simulink library "crm_grc"  (R2024a)
settings: Solver=VariableStepAuto  StartTime=0.0  StopTime=10.0  RelTol=1e-3
undefined symbols (not defined in the file or in its folder): ACRM_Eta_X_rpm, ACRM_MTPAIdGen_X_rpm, ACRM_MTPAIdGen_Y_Nm, ACRM_MTPAIdGenMin_X_rpm, ACRM_MTPAIdGenMin_Y_Nm, ACRM_MTPAIdMot_X_rpm, ACRM_MTPAIdMot_Y_Nm, ACRM_MTPAIdMotMin_X_rpm, ACRM_MTPAIdMotMin_Y_Nm, ACRM_MTPAIqGen_X_rpm, ACRM_MTPAIqGen_Y_Nm, ACRM_MTPAIqGenMin_X_rpm, ACRM_MTPAIqGenMin_Y_Nm, ACRM_MTPAIqMot_X_rpm, ACRM_MTPAIqMot_Y_Nm, ACRM_MTPAIqMotMin_X_rpm, ACRM_MTPAIqMotMin_Y_Nm, ACRM_MTPVIdLimt_X_rpm, DiscIntNeverNeededParam, ENUM_MOTMOD_DISCHARGE, GRC_FAKE_SAMPLE_TIME, KCRM_AtSweep_deg_ovrdflg, KCRM_AtSweep_deg_ovrdval, KCRM_AtSwFWThd_V, KCRM_AtSwStep_ms, KCRM_AtSwThetaStep_deg, KCRM_bRstDebugOverSpd_null, KCRM_BusCurFil_null, KCRM_CurDebugSwt_null, KCRM_CurTqCmdHi_Nm, KCRM_CurTqCmdLo_Nm, KCRM_DcHiBatLDerat_V, KCRM_DcHiBatLLim_V, KCRM_DynoDeratingFiltFac_null, KCRM_FWCEnable_null, KCRM_FWCKi_null, KCRM_FWCKp_null, KCRM_grdIsThetaRampDown_C, KCRM_grdIsThetaRampUp_C, KCRM_IdCmdFilCoeff_null, KCRM_IdCmdMaxLimt_A, KCRM_IdqMapVolHi_V, KCRM_IdqMapVolLo_V, KCRM_IdSp_A_ovrdval, KCRM_IdSpForActvDisc_null, KCRM_IqCmdFilCoeff_null, KCRM_IqDeratingFac_null, KCRM_IqDeratingRecoverTi_ms, KCRM_IqDeratingTi_ms, KCRM_IqDerForFluxWeaken_fac, KCRM_IqSp_A_ovrdval, KCRM_IsSp_A, KCRM_MinVolOfst4FW_V, KCRM_MTPAGenSwitch_flg, KCRM_MTPAMotSwitch_flg, KCRM_MTPVSpdThd_rpm, KCRM_nDebugOverSpd_rpm, KCRM_OCSwFltNormThd_A, KCRM_PILowerLimit_null, KCRM_SpdCtlPrd_s ... (+24)
libraries: GRC_Lib x5, simulink x4
(part 1 of 2)
settings Model: Creator=FVT24180  LastModifiedBy=FVT22063

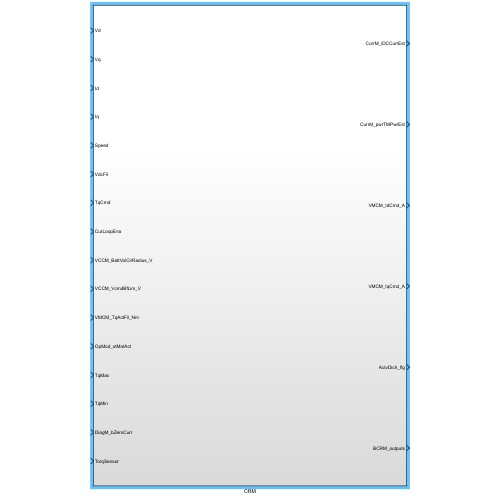
[thumbnail: Simulink's stored preview of the top-level diagram]
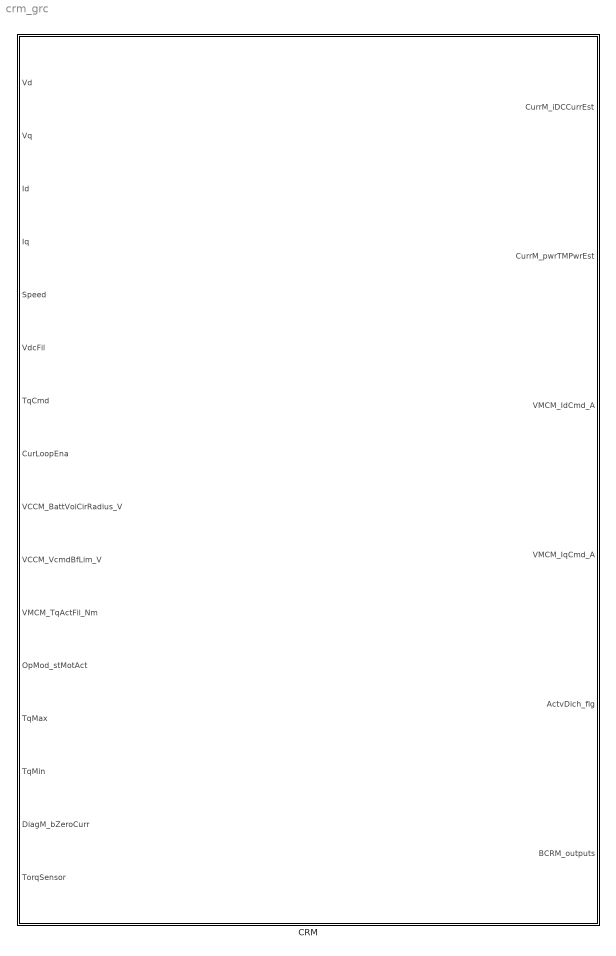
== system crm_grc ==
  CRM : Subsystem

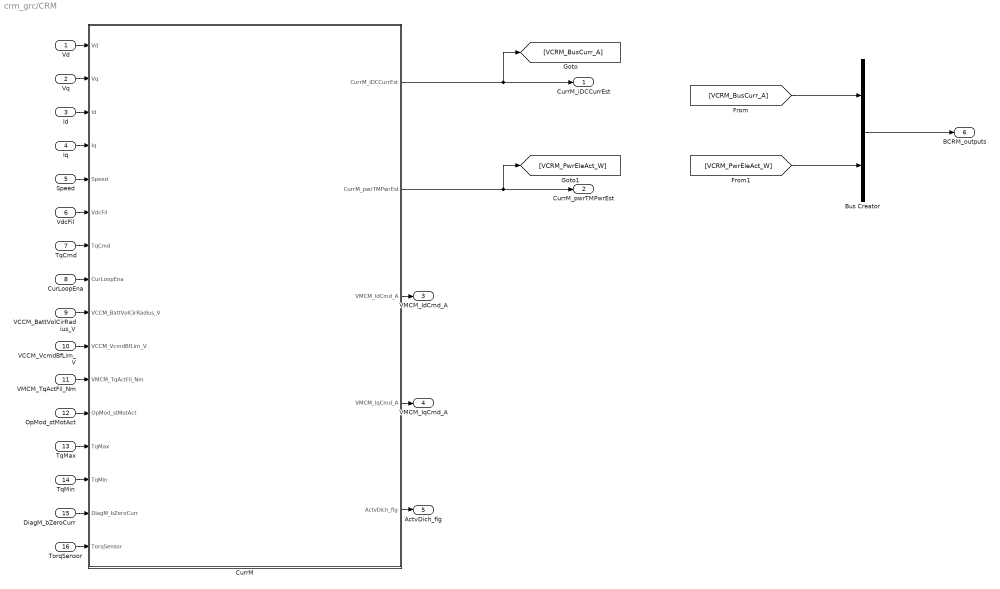
== system crm_grc/CRM ==
  "Vd " : Inport
  "Vq " : Inport  Port=2
  "Id " : Inport  Port=3
  Iq : Inport  Port=4
  "Speed " : Inport  Port=5
  "VdcFil " : Inport  Port=6
  TqCmd : Inport  Port=7
  CurLoopEna : Inport  Port=8
  VCCM_BattVolCirRadius_V : Inport  Port=9
  VCCM_VcmdBfLim_V : Inport  Port=10
  VMCM_TqActFil_Nm : Inport  Port=11
  OpMod_stMotAct : Inport  Port=12
  TqMax : Inport  Port=13
  TqMin : Inport  Port=14
  DiagM_bZeroCurr : Inport  Port=15
  "TorqSensor " : Inport  Port=16
  Bus Creator : BusCreator  Inputs=2  OutDataTypeStr=Bus: BCRM_outputs  NonVirtualBus=on
  CurrM : Subsystem
  CurrM_iDCCurrEst : Outport
  CurrM_pwrTMPwrEst : Outport  Port=2
  VMCM_IdCmd_A : Outport  Port=3
  VMCM_IqCmd_A : Outport  Port=4
  ActvDich_flg : Outport  Port=5
  BCRM_outputs : Outport  Port=6  OutDataTypeStr=Bus: BCRM_outputs
  wires:
  "Vd "/1 -> CurrM/1("Vd ")
  "Speed "/1 -> CurrM/5("Speed ")
  "Vq "/1 -> CurrM/2("Vq ")
  VCCM_VcmdBfLim_V/1 -> CurrM/10(VCCM_VcmdBfLim_V)
  CurLoopEna/1 -> CurrM/8(CurLoopEna)
  Iq/1 -> CurrM/4(Iq)
  TqMin/1 -> CurrM/14(TqMin)
  "VdcFil "/1 -> CurrM/6("VdcFil ")
  "Id "/1 -> CurrM/3("Id ")
  VMCM_TqActFil_Nm/1 -> CurrM/11(VMCM_TqActFil_Nm)
  OpMod_stMotAct/1 -> CurrM/12(OpMod_stMotAct)
  TqCmd/1 -> CurrM/7(TqCmd)
  VCCM_BattVolCirRadius_V/1 -> CurrM/9(VCCM_BattVolCirRadius_V)
  TqMax/1 -> CurrM/13(TqMax)
  CurrM/5(ActvDich_flg) -> ActvDich_flg/1
  "TorqSensor "/1 -> CurrM/16("TorqSensor ")
  DiagM_bZeroCurr/1 -> CurrM/15(DiagM_bZeroCurr)
  CurrM/4(VMCM_IqCmd_A) -> VMCM_IqCmd_A/1
  CurrM/3(VMCM_IdCmd_A) -> VMCM_IdCmd_A/1
  CurrM/1(CurrM_iDCCurrEst) -> [VCRM_BusCurr_A], CurrM_iDCCurrEst/1
  CurrM/2(CurrM_pwrTMPwrEst) -> [VCRM_PwrEleAct_W], CurrM_pwrTMPwrEst/1
  [VCRM_PwrEleAct_W] -> Bus Creator/2
  [VCRM_BusCurr_A] -> Bus Creator/1
  Bus Creator/1 -> BCRM_outputs/1

== system crm_grc/CRM/CurrM ==
  "Vd " : Inport
  "Vq " : Inport  Port=2
  "Id " : Inport  Port=3
  Iq : Inport  Port=4
  "Speed " : Inport  Port=5
  "VdcFil " : Inport  Port=6
  TqCmd : Inport  Port=7
  CurLoopEna : Inport  Port=8
  VCCM_BattVolCirRadius_V : Inport  Port=9
  VCCM_VcmdBfLim_V : Inport  Port=10
  VMCM_TqActFil_Nm : Inport  Port=11
  OpMod_stMotAct : Inport  Port=12
  TqMax : Inport  Port=13
  TqMin : Inport  Port=14
  DiagM_bZeroCurr : Inport  Port=15
  "TorqSensor " : Inport  Port=16
  EstiFun : Subsystem
  MCM : Subsystem
  CurrM_iDCCurrEst : Outport
  CurrM_pwrTMPwrEst : Outport  Port=2
  VMCM_IdCmd_A : Outport  Port=3
  VMCM_IqCmd_A : Outport  Port=4
  ActvDich_flg : Outport  Port=5
  wires:
  Iq/1 -> EstiFun/4(Iq)
  EstiFun/2(VCRM_PwrEleAct_W) -> CurrM_pwrTMPwrEst/1
  VMCM_TqActFil_Nm/1 -> MCM/6(VMCM_TqActFil_Nm)
  VCCM_BattVolCirRadius_V/1 -> MCM/4(VCCM_BattVolCirRadius_V)
  OpMod_stMotAct/1 -> MCM/7(OpMod_stMotAct)
  "Vd "/1 -> EstiFun/1("Vd ")
  CurLoopEna/1 -> MCM/3(CurLoopEna)
  "VdcFil "/1 -> EstiFun/6("VdcFil ")
  VCCM_VcmdBfLim_V/1 -> MCM/5(VCCM_VcmdBfLim_V)
  DiagM_bZeroCurr/1 -> MCM/10(DiagM_bZeroCurr)
  TqMin/1 -> MCM/9(TqMin)
  "TorqSensor "/1 -> MCM/11("TorqSensor ")
  TqMax/1 -> MCM/8(TqMax)
  TqCmd/1 -> MCM/1(TqCmd)
  MCM/2(VMCM_IqCmd_A) -> VMCM_IqCmd_A/1  "VMCM_IqCmd_A"
  MCM/3(ActvDich_flg) -> ActvDich_flg/1  "ActvDich_flg"
  MCM/1(VMCM_IdCmd_A) -> VMCM_IdCmd_A/1  "VMCM_IdCmd_A"
  "Vq "/1 -> EstiFun/2("Vq ")
  "Id "/1 -> EstiFun/3("Id ")
  "Speed "/1 -> MCM/2(SpdFb), EstiFun/5("Speed ")
  EstiFun/1(VCRM_BusCurr_A) -> CurrM_iDCCurrEst/1

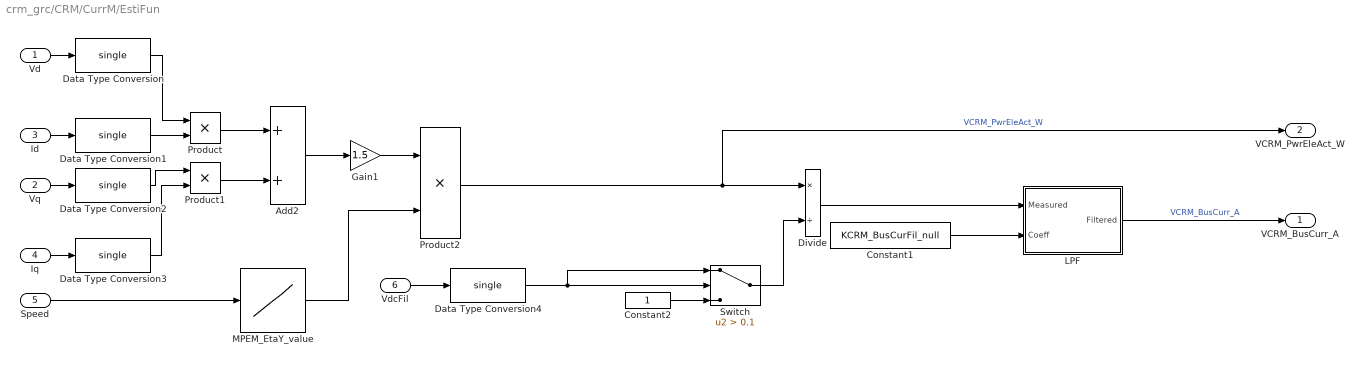
== system crm_grc/CRM/CurrM/EstiFun ==
  "Vd " : Inport
  "Vq " : Inport  Port=2
  "Id " : Inport  Port=3
  Iq : Inport  Port=4
  "Speed " : Inport  Port=5
  "VdcFil " : Inport  Port=6
  Add2 : Sum
  Constant1 : Constant  Value=KCRM_BusCurFil_null
  Constant2 : Constant  OutDataTypeStr=Inherit: Inherit via back propagation
  Data Type Conversion{,1..4} (5 alike) : DataTypeConversion  OutDataTypeStr=single  SaturateOnIntegerOverflow=off  RndMeth=Floor
  Divide : Product  Inputs=*/
  Gain1 : Gain  Gain=1.5  OutDataTypeStr=Inherit: Same as input
  "LPF " : Subsystem
  MPEM_EtaY_value : Lookup_n-D  NumberOfTableDimensions=1  BreakpointsForDimension1=ACRM_Eta_X_rpm  Table=MCRM_Eta_Y_null  ExtrapMethod=Clip  UseLastTableValue=on  InternalRulePriority=Speed  RndMeth=Simplest
  Product : Product  OutDataTypeStr=Inherit: Same as first input
  Product1 : Product  OutDataTypeStr=Inherit: Same as first input
  Product2 : Product  OutDataTypeStr=Inherit: Same as first input
  Switch : Switch  Criteria=u2 > Threshold  Threshold=0.1  SaturateOnIntegerOverflow=off  InputSameDT=off
  VCRM_BusCurr_A : Outport  VectorParamsAs1DForOutWhenUnconnected=off
  VCRM_PwrEleAct_W : Outport  Port=2  VectorParamsAs1DForOutWhenUnconnected=off
  wires:
  "Vd "/1 -> Data Type Conversion/1
  "Id "/1 -> Data Type Conversion1/1
  "Vq "/1 -> Data Type Conversion2/1
  Iq/1 -> Data Type Conversion3/1
  Product1/1 -> Add2/2
  Product/1 -> Add2/1
  Add2/1 -> Gain1/1
  "Speed "/1 -> MPEM_EtaY_value/1
  MPEM_EtaY_value/1 -> Product2/2
  Product2/1 -> Divide/1, VCRM_PwrEleAct_W/1  "VCRM_PwrEleAct_W"
  Divide/1 -> "LPF "/1(Measured)
  "LPF "/1(Filtered) -> VCRM_BusCurr_A/1  "VCRM_BusCurr_A"
  Gain1/1 -> Product2/1
  Constant1/1 -> "LPF "/2("Coeff ")
  "VdcFil "/1 -> Data Type Conversion4/1
  Switch/1 -> Divide/2
  Constant2/1 -> Switch/3
  Data Type Conversion/1 -> Product/1
  Data Type Conversion1/1 -> Product/2
  Data Type Conversion2/1 -> Product1/1
  Data Type Conversion3/1 -> Product1/2
  Data Type Conversion4/1 -> Switch/1, Switch/2

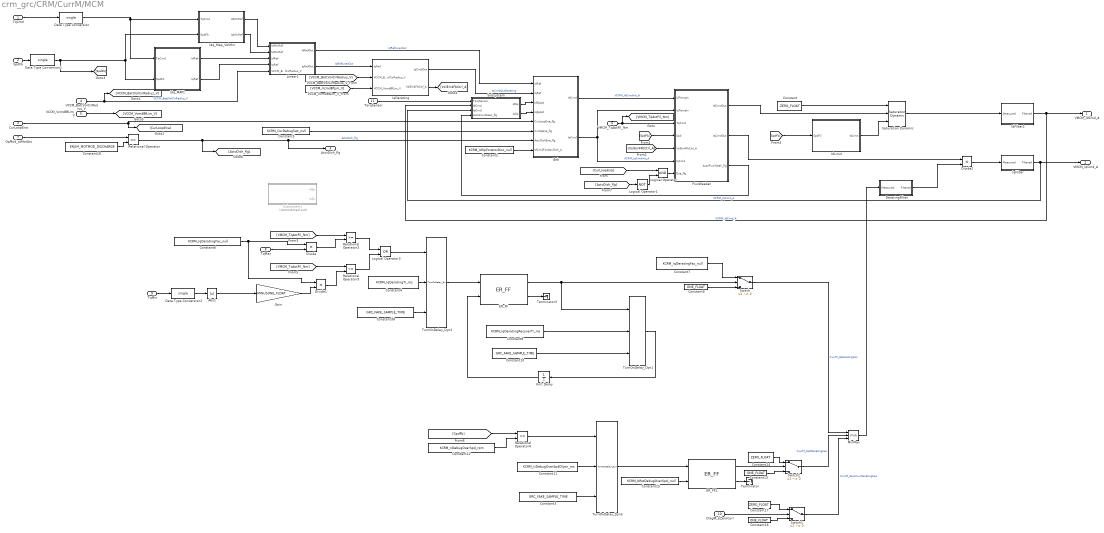
== system crm_grc/CRM/CurrM/MCM ==
  TqCmd : Inport
  SpdFb : Inport  Port=2
  CurLoopEna : Inport  Port=3
  VCCM_BattVolCirRadius_V : Inport  Port=4
  VCCM_VcmdBfLim_V : Inport  Port=5
  VMCM_TqActFil_Nm : Inport  Port=6
  OpMod_stMotAct : Inport  Port=7
  TqMax : Inport  Port=8
  TqMin : Inport  Port=9
  DiagM_bZeroCurr : Inport  Port=10
  "TorqSensor " : Inport  Port=11
  Abs1 : Abs  SaturateOnIntegerOverflow=off
  Constant : Constant  Value=ZERO_FLOAT
  Constant10 : Constant  Value=GRC_FAKE_SAMPLE_TIME
  Constant11 : Constant  Value=KCRM_tiDebugOverSpdDlyon_ms  OutDataTypeStr=single
  Constant12 : Constant  Value=KCRM_nDebugOverSpd_rpm  OutDataTypeStr=single
  Constant13 : Constant  Value=ONE_FLOAT  OutDataTypeStr=single
  Constant14 : Constant  Value=ZERO_FLOAT  OutDataTypeStr=single
  Constant15 : Constant  Value=KCRM_bRstDebugOverSpd_null  OutDataTypeStr=single
  Constant16 : Constant  Value=ONE_FLOAT  OutDataTypeStr=single
  Constant17 : Constant  Value=ZERO_FLOAT  OutDataTypeStr=single
  Constant18 : Constant  Value=ENUM_MOTMOD_DISCHARGE
  Constant2 : Constant  Value=KCRM_IdSpForActvDisc_null  OutDataTypeStr=single
  Constant3 : Constant  Value=GRC_FAKE_SAMPLE_TIME
  Constant38 : Constant  Value=GRC_FAKE_SAMPLE_TIME
  Constant4 : Constant  Value=KCRM_IqDeratingTi_ms  OutDataTypeStr=single
  Constant5 : Constant  Value=KCRM_CurDebugSwt_null  OutDataTypeStr=boolean
  Constant6 : Constant  Value=KCRM_IqDeratingFac_null  OutDataTypeStr=single
  Constant7 : Constant  Value=KCRM_IqDeratingFac_null  OutDataTypeStr=single
  Constant8 : Constant  Value=KCRM_IqDeratingRecoverTi_ms  OutDataTypeStr=single
  Constant9 : Constant  Value=ONE_FLOAT  OutDataTypeStr=single
  Data Type Conversion : DataTypeConversion  OutDataTypeStr=single  SaturateOnIntegerOverflow=off  RndMeth=Floor
  Data Type Conversion1 : DataTypeConversion  OutDataTypeStr=single  SaturateOnIntegerOverflow=off  RndMeth=Floor
  Data Type Conversion2 : DataTypeConversion  OutDataTypeStr=single  SaturateOnIntegerOverflow=off  RndMeth=Floor
  DeratingFilter : Subsystem
  Divide : Product  Inputs=**
  Divide1 : Product  Inputs=**
  Divide2 : Product  Inputs=**
  ER_FF : GRC_Lib/Memory/ER_FF  FalseVal=0  TrueVal=1
  ER_FF1 : GRC_Lib/Memory/ER_FF  FalseVal=0  TrueVal=1
  "FluxWeaken " : Subsystem
  Gain : Gain  Gain=MINUSONE_FLOAT
  IArb : Stateflow chart  TreatAsAtomicUnit=on
  IdFilter2 : Subsystem
  IdLimit : Subsystem
  Idq_MAP1 : Subsystem
  Idq_Map_VolMin : Subsystem
  IqDerating : Subsystem
  IqFilter : Subsystem
  Linear1 : Subsystem
  Logical Operator : Logic  AllPortsSameDT=off  OutDataTypeStr=boolean
  Logical Operator1 : Logic  Operator=NOT  AllPortsSameDT=off  OutDataTypeStr=boolean
  Logical Operator3 : Logic  Operator=OR  AllPortsSameDT=off  OutDataTypeStr=boolean
  MinMax : MinMax  Inputs=3
  Relational Operator : RelationalOperator  Operator===  OutDataTypeStr=boolean  InputSameDT=off
  Relational Operator2 : RelationalOperator  OutDataTypeStr=boolean  RndMeth=Simplest  InputSameDT=off
  Relational Operator3 : RelationalOperator  Operator=<=  OutDataTypeStr=boolean  RndMeth=Simplest  InputSameDT=off
  Relational Operator4 : RelationalOperator  OutDataTypeStr=boolean  RndMeth=Simplest  InputSameDT=off
  Saturation Dynamic : simulink/Discontinuities/Saturation Dynamic  OutMin=[]  OutMax=[]  OutDataTypeStr=Inherit: Same as second input  OutDataType=fixdt(1, 16)  OutScaling=2^-10  DoSatur=off
  Subsystem : Subsystem
  Subsystem1 : Subsystem  Commented=on
  Switch : Switch  Criteria=u2 ~= 0  SaturateOnIntegerOverflow=off  InputSameDT=off
  Switch1 : Switch  Criteria=u2 ~= 0  SaturateOnIntegerOverflow=off  InputSameDT=off
  Switch2 : Switch  Criteria=u2 ~= 0  SaturateOnIntegerOverflow=off  InputSameDT=off
  Terminator : Terminator
  Terminator3 : Terminator
  TurnOnDelay_Dyn1 : GRC_Lib/Delay/TurnOnDelay_Dyn  IpDT=single
  TurnOnDelay_Dyn2 : GRC_Lib/Delay/TurnOnDelay_Dyn  IpDT=single
  TurnOnDelay_Dyn3 : GRC_Lib/Delay/TurnOnDelay_Dyn  IpDT=single
  Unit Delay : UnitDelay  SampleTime=-1
  VMCM_IdCmd_A : Outport
  VMCM_IqCmd_A : Outport  Port=2
  ActvDich_flg : Outport  Port=3
  wires:
  TqCmd/1 -> Data Type Conversion/1
  VCCM_BattVolCirRadius_V/1 -> Linear1/5(VCCM_BattVolCirRadius_V), [VCCM_BattVolCirRadius_V]  "VCCM_BattVolCirRadius_V"
  Constant2/1 -> IArb/8(IdCmdForActvDich_A)
  IqFilter/1(Filtered) -> Subsystem/3("IqCmd "), VMCM_IqCmd_A/1  "VCRM_IqCmd_A"
  IdFilter2/1(Filtered) -> Subsystem/2("IdCmd "), VMCM_IdCmd_A/1  "VCRM_IdCmd_A"
  CurLoopEna/1 -> IArb/5(CurLoopEna_flg), [CurLoopEna]
  SpdFb/1 -> Data Type Conversion1/1
  Constant5/1 -> IArb/6(CurSpEna_flg)
  Subsystem/1(IdSp) -> IArb/3(IdSpAct)
  Subsystem/2(IqSp) -> IArb/4(IqSpAct)
  Idq_MAP1/1(IdRef) -> Linear1/3(IdRef)
  Idq_MAP1/2(IqRef) -> Linear1/4(IqRef)
  [VCCM_BattVolCirRadius_V] -> IqDerating/2(VCCM_BattVolCirRadius_V)
  [VCCM_VcmdBfLim_V] -> IqDerating/3(VCCM_VcmdBfLim_V)
  Linear1/2(IqRefOut) -> IqDerating/1(IqRef)  "IqRefLinerOut"
  IqDerating/1(IqCmdOut) -> IArb/2(IqRef)  "IqCmdOutDerating"
  Linear1/1(IdRefOut) -> IArb/1(IdRef)  "IdRefLinerOut"
  IArb/1(IdCmd) -> "FluxWeaken "/1("IdTempIn ")  "VCRM_IdCmdinit_A"
  IArb/2(IqCmd) -> "FluxWeaken "/2("IqTempIn "), "FluxWeaken "/6("IqCmd ")  "VCRM_IqCmdinit_A"
  "FluxWeaken "/2("IqCmdOut ") -> Divide2/1
  Saturation Dynamic/1 -> IdFilter2/1(Measured)
  "FluxWeaken "/1(IdCmdOut) -> Saturation Dynamic/2
  Constant/1 -> Saturation Dynamic/1
  VMCM_TqActFil_Nm/1 -> [VMCM_TqActFil_Nm], "FluxWeaken "/3(TqCmd)
  IdLimit/1("IdLimit ") -> Saturation Dynamic/3
  [SpdFb] -> IdLimit/1("SpdFil ")
  Relational Operator/1 -> [ActvDich_flg], IArb/7(ActvDichEna_flg), ActvDich_flg/1  "ActvDich_flg"
  Constant18/1 -> Relational Operator/2
  OpMod_stMotAct/1 -> Relational Operator/1
  [SpdFb] -> "FluxWeaken "/4(Spd)
  [VolErr4FbCtrl_A] -> "FluxWeaken "/5(VolErr4FbCtrl_A)
  [CurLoopEna] -> Logical Operator/1
  VCCM_VcmdBfLim_V/1 -> [VCCM_VcmdBfLim_V]
  ER_FF/2 -> Terminator3/1
  Gain/1 -> Divide1/2
  Relational Operator2/1 -> Logical Operator3/1
  Abs1/1 -> Gain/1
  MinMax/1 -> DeratingFilter/1(Measured)
  Constant6/1 -> Divide1/1, Divide/1
  Logical Operator3/1 -> TurnOnDelay_Dyn2/1
  TurnOnDelay_Dyn1/1 -> Unit Delay/1
  Relational Operator3/1 -> Logical Operator3/2
  Constant7/1 -> Switch/1
  Constant9/1 -> Switch/3
  TqMax/1 -> Divide/2
  Divide1/1 -> Relational Operator3/2
  Divide/1 -> Relational Operator2/2
  TqMin/1 -> Data Type Conversion2/1
  ER_FF/1 -> Switch/2, TurnOnDelay_Dyn1/1
  Divide2/1 -> IqFilter/1(Measured)
  Constant4/1 -> TurnOnDelay_Dyn2/2
  Constant38/1 -> TurnOnDelay_Dyn2/3
  TurnOnDelay_Dyn2/1 -> ER_FF/1
  Constant10/1 -> TurnOnDelay_Dyn1/3
  Constant8/1 -> TurnOnDelay_Dyn1/2
  Unit Delay/1 -> ER_FF/2
  [VMCM_TqActFil_Nm] -> Relational Operator2/1
  [VMCM_TqActFil_Nm] -> Relational Operator3/1
  [SpdFb] -> Relational Operator4/1
  Relational Operator4/1 -> TurnOnDelay_Dyn3/1
  Constant13/1 -> Switch2/3
  Constant14/1 -> Switch2/1
  Constant12/1 -> Relational Operator4/2
  Constant3/1 -> TurnOnDelay_Dyn3/3
  Constant11/1 -> TurnOnDelay_Dyn3/2
  TurnOnDelay_Dyn3/1 -> ER_FF1/1
  ER_FF1/1 -> Switch2/2
  Constant15/1 -> ER_FF1/2
  Switch/1 -> MinMax/1  "CurrM_IqDeratingFac"
  Switch2/1 -> MinMax/2  "CurrM_SpdDeratingFac"
  ER_FF1/2 -> Terminator/1
  DeratingFilter/1(Filtered) -> Divide2/2
  [ActvDich_flg] -> Logical Operator1/1
  Logical Operator1/1 -> Logical Operator/2
  Logical Operator/1 -> "FluxWeaken "/7(Ena_flg)
  DiagM_bZeroCurr/1 -> Switch1/2
  Constant17/1 -> Switch1/1
  Constant16/1 -> Switch1/3
  Switch1/1 -> MinMax/3  "CurrM_ZeroCurrDeratingFac"
  "TorqSensor "/1 -> Subsystem/1("TorqSensor ")
  IqDerating/2(VolErr4FbCtrl_A) -> [VolErr4FbCtrl_A]
  "FluxWeaken "/3("AutoFluxWeak_flg ") -> Subsystem/4("AutoFluxWeak_flg ")
  Data Type Conversion/1 -> Idq_Map_VolMin/1(TqCmd), Idq_MAP1/1(TqCmd)
  Data Type Conversion1/1 -> [SpdFb], Idq_Map_VolMin/2(SpdFb), Idq_MAP1/2(SpdFb)
  Data Type Conversion2/1 -> Abs1/1
  Idq_Map_VolMin/1(IdMinRef) -> Linear1/1(IdMinRef)
  Idq_Map_VolMin/2(IqMinRef) -> Linear1/2(IqMinRef)

== system crm_grc/CRM/CurrM/EstiFun/LPF  ==
  Measured : Inport  PortDimensions=1
  "Coeff " : Inport  Port=2  PortDimensions=1
  Add : Sum
  Product : Product  RndMeth=Zero
  Subtract : Sum  Inputs=+-
  Unit Delay : UnitDelay  SampleTime=-1
  Filtered : Outport
  wires:
  Measured/1 -> Subtract/1
  Unit Delay/1 -> Subtract/2, Add/2
  Subtract/1 -> Product/1
  Product/1 -> Add/1
  Add/1 -> Filtered/1, Unit Delay/1
  "Coeff "/1 -> Product/2

== system crm_grc/CRM/CurrM/MCM/DeratingFilter ==
  note: Description:
      | 1 order low pass filter. The constant value depends on the cut-off frequency,
  Measured : Inport  PortDimensions=1
  Add : Sum
  Constant : Constant  Value=KCRM_DynoDeratingFiltFac_null  OutDataTypeStr=single
  Product : Product  RndMeth=Zero
  Subtract : Sum  Inputs=+-
  Unit Delay : UnitDelay  SampleTime=-1
  Filtered : Outport
  wires:
  Measured/1 -> Subtract/1
  Unit Delay/1 -> Subtract/2, Add/2
  Subtract/1 -> Product/1
  Constant/1 -> Product/2
  Product/1 -> Add/1
  Add/1 -> Filtered/1, Unit Delay/1

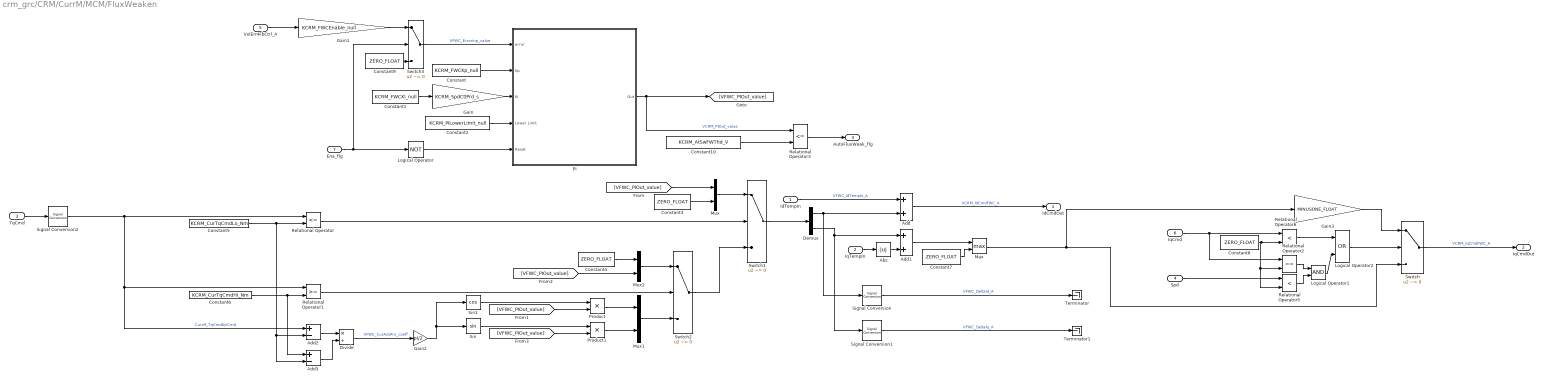
== system crm_grc/CRM/CurrM/MCM/FluxWeaken  ==
  "IdTempIn " : Inport
  "IqTempIn " : Inport  Port=2
  TqCmd : Inport  Port=3
  Spd : Inport  Port=4
  VolErr4FbCtrl_A : Inport  Port=5
  "IqCmd " : Inport  Port=6
  Ena_flg : Inport  Port=7
  Abs : Abs  SaturateOnIntegerOverflow=off
  Add : Sum  OutDataTypeStr=Inherit: Same as first input
  Add1 : Sum  OutDataTypeStr=Inherit: Same as first input
  Add2 : Sum  Inputs=+-  OutDataTypeStr=Inherit: Same as first input
  Add3 : Sum  Inputs=+-  OutDataTypeStr=Inherit: Same as first input
  Constant : Constant  Value=KCRM_FWCKp_null
  Constant1 : Constant  Value=KCRM_FWCKi_null
  Constant10 : Constant  Value=KCRM_AtSwFWThd_V
  Constant2 : Constant  Value=KCRM_PILowerLimit_null
  Constant{3..4,7..9} (5 alike) : Constant  Value=ZERO_FLOAT  OutDataTypeStr=single
  Constant5 : Constant  Value=KCRM_CurTqCmdLo_Nm
  Constant6 : Constant  Value=KCRM_CurTqCmdHi_Nm
  Demux : Demux  Outputs=2
  Divide : Product  Inputs=*/  OutDataTypeStr=Inherit: Same as first input
  Gain : Gain  Gain=KCRM_SpdCtlPrd_s
  Gain1 : Gain  Gain=KCRM_FWCEnable_null  OutDataTypeStr=Inherit: Inherit via back propagation
  Gain2 : Gain  Gain=pi/2  OutDataTypeStr=Inherit: Same as input
  Gain3 : Gain  Gain=MINUSONE_FLOAT
  Logical Operator : Logic  Operator=NOT  AllPortsSameDT=off  OutDataTypeStr=boolean
  Logical Operator1 : Logic  AllPortsSameDT=off  OutDataTypeStr=boolean
  Logical Operator2 : Logic  Operator=OR  AllPortsSameDT=off  OutDataTypeStr=boolean
  Max : MinMax  Function=max  Inputs=2  OutDataTypeStr=Inherit: Inherit via back propagation
  Mux : Mux  Inputs=2
  Mux1 : Mux  Inputs=2
  Mux2 : Mux  Inputs=2
  "PI " : Subsystem
  Product : Product
  Product1 : Product
  Relational Operator : RelationalOperator  Operator=<=  OutDataTypeStr=boolean  RndMeth=Simplest  InputSameDT=off
  Relational Operator1 : RelationalOperator  OutDataTypeStr=boolean  RndMeth=Simplest  InputSameDT=off
  Relational Operator2 : RelationalOperator  Operator===  OutDataTypeStr=boolean  InputSameDT=off
  Relational Operator3 : RelationalOperator  Operator=<=  OutDataTypeStr=boolean  RndMeth=Simplest  InputSameDT=off
  Relational Operator5 : RelationalOperator  Operator=<  OutDataTypeStr=boolean  InputSameDT=off
  Relational Operator6 : RelationalOperator  Operator=<  OutDataTypeStr=boolean  InputSameDT=off
  Signal Conversion : SignalConversion  OverrideOpt=off
  Signal Conversion1 : SignalConversion  OverrideOpt=off
  Signal Conversion2 : SignalConversion  OverrideOpt=off
  Sin : Trigonometry
  Sin1 : Trigonometry  Operator=cos
  Switch : Switch  Criteria=u2 ~= 0  SaturateOnIntegerOverflow=off  InputSameDT=off
  Switch1 : Switch  Criteria=u2 ~= 0  OutDataTypeStr=Inherit: Inherit via back propagation  SaturateOnIntegerOverflow=off  InputSameDT=off
  Switch2 : Switch  Criteria=u2 ~= 0  OutDataTypeStr=Inherit: Inherit via back propagation  SaturateOnIntegerOverflow=off  InputSameDT=off
  Switch3 : Switch  Criteria=u2 ~= 0  SaturateOnIntegerOverflow=off  InputSameDT=off
  Terminator : Terminator
  Terminator1 : Terminator
  IdCmdOut : Outport  VectorParamsAs1DForOutWhenUnconnected=off
  "IqCmdOut " : Outport  Port=2  VectorParamsAs1DForOutWhenUnconnected=off
  "AutoFluxWeak_flg " : Outport  Port=3  VectorParamsAs1DForOutWhenUnconnected=off
  wires:
  Constant/1 -> "PI "/2(Kp)
  Constant1/1 -> Gain/1
  Constant2/1 -> "PI "/4(Lower Limit)
  Ena_flg/1 -> Logical Operator/1, Switch3/2
  "PI "/1(Out) -> Relational Operator3/1, [VFWC_PIOut_value]  "VCRM_PIOut_value"
  Mux/1 -> Switch1/1
  [VFWC_PIOut_value] -> Mux/1
  Constant3/1 -> Mux/2
  Switch2/1 -> Switch1/3
  Constant4/1 -> Mux2/1
  [VFWC_PIOut_value] -> Mux2/2
  Mux2/1 -> Switch2/1
  Switch1/1 -> Demux/1
  "IdTempIn "/1 -> Add/1  "VFWC_IdTempIn_A"
  Demux/1 -> Signal Conversion/1, Add/2
  "IqTempIn "/1 -> Abs/1
  Demux/2 -> Add1/1, Signal Conversion1/1
  Add/1 -> IdCmdOut/1  "VCRM_IdCmdFWC_A"
  Signal Conversion/1 -> Terminator/1  "VFWC_DeltaId_A"
  Signal Conversion1/1 -> Terminator1/1  "VFWC_DeltaIq_A"
  Mux1/1 -> Switch2/3
  Constant5/1 -> Add3/2, Add2/2, Relational Operator/2
  Constant6/1 -> Add3/1, Relational Operator1/2
  Relational Operator/1 -> Switch1/2
  Relational Operator1/1 -> Switch2/2
  Add2/1 -> Divide/1
  Add3/1 -> Divide/2
  [VFWC_PIOut_value] -> Product/2
  Sin1/1 -> Product/1
  Sin/1 -> Product1/1
  [VFWC_PIOut_value] -> Product1/2
  Product/1 -> Mux1/1
  Product1/1 -> Mux1/2
  Divide/1 -> Gain2/1  "VFWC_CurAssPro_coeff"
  Gain2/1 -> Sin/1, Sin1/1
  Constant7/1 -> Max/2
  Add1/1 -> Max/1
  Logical Operator/1 -> "PI "/5("Reset ")
  Gain3/1 -> Switch/1
  Relational Operator6/1 -> Logical Operator2/1
  Relational Operator5/1 -> Logical Operator1/2
  Logical Operator2/1 -> Switch/2
  Logical Operator1/1 -> Logical Operator2/2
  Relational Operator2/1 -> Logical Operator1/1
  Switch/1 -> "IqCmdOut "/1  "VCRM_IqCmdFWC_A"
  "IqCmd "/1 -> Relational Operator2/1, Relational Operator6/1
  Constant8/1 -> Relational Operator5/2, Relational Operator2/2, Relational Operator6/2
  Spd/1 -> Relational Operator5/1
  Max/1 -> Switch/3, Gain3/1
  VolErr4FbCtrl_A/1 -> Gain1/1
  TqCmd/1 -> Signal Conversion2/1
  Switch3/1 -> "PI "/1(error)  "VFWC_ErrorInp_value"
  Gain1/1 -> Switch3/1
  Constant9/1 -> Switch3/3
  Abs/1 -> Add1/2
  Signal Conversion2/1 -> Relational Operator/1, Add2/1, Relational Operator1/1  "CurrM_TqCmdbyICmd"
  Relational Operator3/1 -> "AutoFluxWeak_flg "/1
  Constant10/1 -> Relational Operator3/2
  Gain/1 -> "PI "/3(Ki)

== system crm_grc/CRM/CurrM/MCM/IdFilter2 ==
  note: Description:
      | 1 order low pass filter. The constant value depends on the cut-off frequency,
  Measured : Inport  PortDimensions=1
  Add : Sum
  Constant : Constant  Value=KCRM_IdCmdFilCoeff_null  OutDataTypeStr=single
  Product : Product  RndMeth=Zero
  Subtract : Sum  Inputs=+-
  Unit Delay : UnitDelay  SampleTime=-1
  Filtered : Outport
  wires:
  Add/1 -> Filtered/1, Unit Delay/1
  Product/1 -> Add/1
  Subtract/1 -> Product/1
  Measured/1 -> Subtract/1
  Unit Delay/1 -> Add/2, Subtract/2
  Constant/1 -> Product/2

== system crm_grc/CRM/CurrM/MCM/IdLimit ==
  note: 额定
  "SpdFil " : Inport
  1-D Lookup Table : Lookup_n-D  NumberOfTableDimensions=1  BreakpointsForDimension1=ACRM_MTPVIdLimt_X_rpm  Table=MCRM_MTPVIdLimt_Y_A  ExtrapMethod=Clip  UseLastTableValue=on  InternalRulePriority=Speed  RndMeth=Simplest
  Constant : Constant  Value=KCRM_MTPVSpdThd_rpm
  Constant3 : Constant  Value=KCRM_IdCmdMaxLimt_A  VectorParams1D=off  SampleTime=-1
  Relational Operator : RelationalOperator  Operator=>  OutDataTypeStr=boolean  RndMeth=Simplest  InputSameDT=off
  Switch : Switch  Criteria=u2 ~= 0  SaturateOnIntegerOverflow=off  InputSameDT=off
  "IdLimit " : Outport  VectorParamsAs1DForOutWhenUnconnected=off
  wires:
  Switch/1 -> "IdLimit "/1
  "SpdFil "/1 -> 1-D Lookup Table/1, Relational Operator/1
  Constant/1 -> Relational Operator/2
  Constant3/1 -> Switch/3
  Relational Operator/1 -> Switch/2
  1-D Lookup Table/1 -> Switch/1

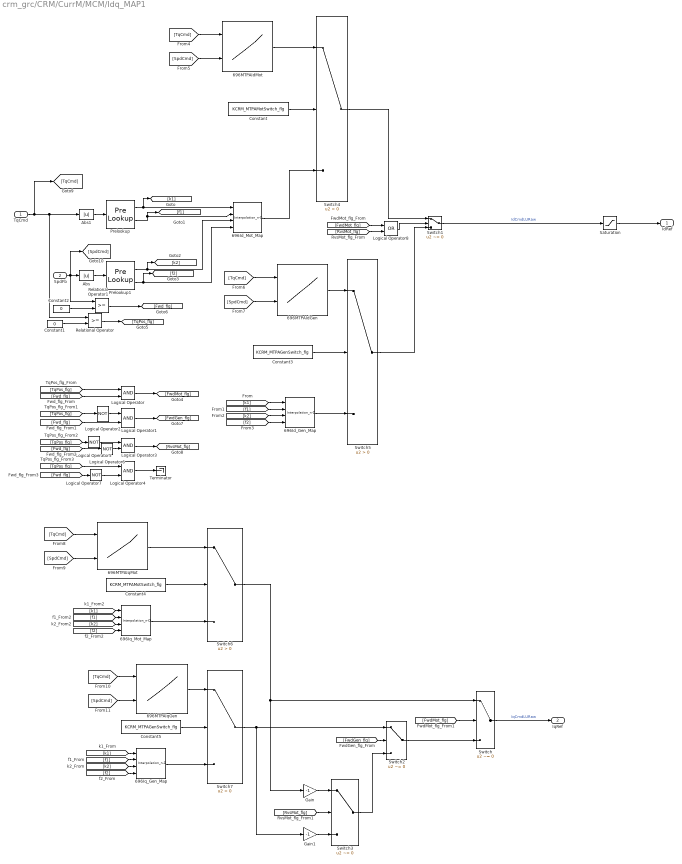
== system crm_grc/CRM/CurrM/MCM/Idq_MAP1 ==
  TqCmd : Inport
  SpdFb : Inport  Port=2
  696Id_Gen_Map : Interpolation_n-D  Table=MCRM_MTPAIdGen_Z_A
  696Id_Mot_Map : Interpolation_n-D  Table=MCRM_MTPAIdMot_Z_A
  696Iq_Gen_Map : Interpolation_n-D  Table=MCRM_MTPAIqGen_Z_A
  696Iq_Mot_Map : Interpolation_n-D  Table=MCRM_MTPAIqMot_Z_A
  696MTPAIdGen : Lookup_n-D  BreakpointsForDimension1=ACRM_MTPAIdGen_Y_Nm  BreakpointsForDimension2=ACRM_MTPAIdGen_X_rpm  Table=MCRM_MTPAIdGen_Z_A  InternalRulePriority=Speed  RndMeth=Simplest
      settings: InputPortMap=u0,u1
  696MTPAIdMot : Lookup_n-D  BreakpointsForDimension1=ACRM_MTPAIdMot_Y_Nm  BreakpointsForDimension2=ACRM_MTPAIdMot_X_rpm  Table=MCRM_MTPAIdMot_Z_A  InternalRulePriority=Speed  RndMeth=Simplest
      settings: InputPortMap=u0,u1
  696MTPAIqGen : Lookup_n-D  BreakpointsForDimension1=ACRM_MTPAIqGen_Y_Nm  BreakpointsForDimension2=ACRM_MTPAIqGen_X_rpm  Table=MCRM_MTPAIqGen_Z_A  InternalRulePriority=Speed  RndMeth=Simplest
      settings: InputPortMap=u0,u1
  696MTPAIqMot : Lookup_n-D  BreakpointsForDimension1=ACRM_MTPAIqMot_Y_Nm  BreakpointsForDimension2=ACRM_MTPAIqMot_X_rpm  Table=MCRM_MTPAIqMot_Z_A  InternalRulePriority=Speed  RndMeth=Simplest
      settings: InputPortMap=u0,u1
  Abs : Abs
  Abs1 : Abs
  Constant : Constant  Value=KCRM_MTPAMotSwitch_flg
  Constant1 : Constant  Value=0  OutDataTypeStr=uint8
  Constant2 : Constant  Value=0  OutDataTypeStr=uint8
  Constant3 : Constant  Value=KCRM_MTPAGenSwitch_flg
  Constant4 : Constant  Value=KCRM_MTPAMotSwitch_flg
  Constant5 : Constant  Value=KCRM_MTPAGenSwitch_flg
  Gain : Gain  Gain=-1
  Gain1 : Gain  Gain=-1
  Logical Operator{,1,3..4} (4 alike) : Logic  AllPortsSameDT=off  OutDataTypeStr=boolean
  Logical Operator{2,5..7} (4 alike) : Logic  Operator=NOT  AllPortsSameDT=off  OutDataTypeStr=boolean
  Logical Operator8 : Logic  Operator=OR  AllPortsSameDT=off  OutDataTypeStr=boolean
  Prelookup : PreLookup  BreakpointsData=ACRM_MTPAIdMot_Y_Nm  ExtrapMethod=Linear
  Prelookup1 : PreLookup  BreakpointsData=ACRM_MTPAIdMot_X_rpm  ExtrapMethod=Linear
  Relational Operator : RelationalOperator  OutDataTypeStr=boolean  InputSameDT=off
  Relational Operator1 : RelationalOperator  OutDataTypeStr=boolean  InputSameDT=off
  Saturation : Saturate  UpperLimit=0  LowerLimit=-500
      settings: AttributesFormatString=%<UpperLimit>\n%<LowerLimit>
  Switch{,1..3} (4 alike) : Switch  Criteria=u2 ~= 0
  Switch{4..7} (4 alike) : Switch  Criteria=u2 > Threshold  SaturateOnIntegerOverflow=off  InputSameDT=off
  Terminator : Terminator
  IdRef : Outport
  IqRef : Outport  Port=2
  wires:
  Constant2/1 -> Relational Operator1/2
  [f2] -> 696Iq_Mot_Map/4
  Relational Operator1/1 -> [Fwd_flg]
  [k1] -> 696Iq_Mot_Map/1
  [Fwd_flg] -> Logical Operator7/1
  696Id_Mot_Map/1 -> Switch4/3
  Prelookup1/2 -> 696Id_Mot_Map/4, [f2]
  [k2] -> 696Iq_Gen_Map/3
  [f1] -> 696Iq_Gen_Map/2
  Logical Operator/1 -> [FwdMot_flg]
  Prelookup1/1 -> 696Id_Mot_Map/3, [k2]
  [k1] -> 696Iq_Gen_Map/1
  [FwdGen_flg] -> Switch2/2
  [f2] -> 696Iq_Gen_Map/4
  [TqPos_flg] -> Logical Operator2/1
  Abs/1 -> Prelookup1/1
  Logical Operator3/1 -> [RvsMot_flg]
  Prelookup/2 -> 696Id_Mot_Map/2, [f1]
  [TqPos_flg] -> Logical Operator/1
  Abs1/1 -> Prelookup/1
  [k2] -> 696Iq_Mot_Map/3
  TqCmd/1 -> [TqCmd], Relational Operator/1, Abs1/1
  Constant1/1 -> Relational Operator/2
  [TqPos_flg] -> Logical Operator5/1
  Logical Operator2/1 -> Logical Operator1/1
  SpdFb/1 -> [SpdCmd], Relational Operator1/1, Abs/1
  [Fwd_flg] -> Logical Operator6/1
  [Fwd_flg] -> Logical Operator/2
  [TqPos_flg] -> Logical Operator4/1
  [Fwd_flg] -> Logical Operator1/2
  Prelookup/1 -> [k1], 696Id_Mot_Map/1
  [RvsMot_flg] -> Logical Operator8/2
  Gain1/1 -> Switch3/3
  [f1] -> 696Iq_Mot_Map/2
  Relational Operator/1 -> [TqPos_flg]
  Logical Operator4/1 -> Terminator/1
  Logical Operator6/1 -> Logical Operator3/2
  Logical Operator5/1 -> Logical Operator3/1
  Logical Operator1/1 -> [FwdGen_flg]
  Switch2/1 -> Switch/3
  Gain/1 -> Switch3/1
  Saturation/1 -> IdRef/1
  [FwdMot_flg] -> Logical Operator8/1
  [FwdMot_flg] -> Switch/2
  Switch1/1 -> Saturation/1  "IdCmdLURaw"
  Switch/1 -> IqRef/1  "IqCmdLURaw"
  Switch3/1 -> Switch2/3
  [RvsMot_flg] -> Switch3/2
  Logical Operator8/1 -> Switch1/2
  Logical Operator7/1 -> Logical Operator4/2
  [k1] -> 696Id_Gen_Map/1
  [f1] -> 696Id_Gen_Map/2
  [k2] -> 696Id_Gen_Map/3
  [f2] -> 696Id_Gen_Map/4
  Constant/1 -> Switch4/2
  [TqCmd] -> 696MTPAIdMot/1
  696MTPAIdMot/1 -> Switch4/1
  [SpdCmd] -> 696MTPAIdMot/2
  Switch4/1 -> Switch1/1
  696Id_Gen_Map/1 -> Switch5/3
  Constant3/1 -> Switch5/2
  696MTPAIdGen/1 -> Switch5/1
  [SpdCmd] -> 696MTPAIdGen/2
  [TqCmd] -> 696MTPAIdGen/1
  [TqCmd] -> 696MTPAIqMot/1
  Constant4/1 -> Switch6/2
  [SpdCmd] -> 696MTPAIqMot/2
  696MTPAIqMot/1 -> Switch6/1
  696Iq_Mot_Map/1 -> Switch6/3
  Switch6/1 -> Gain/1, Switch/1
  [SpdCmd] -> 696MTPAIqGen/2
  696MTPAIqGen/1 -> Switch7/1
  Constant5/1 -> Switch7/2
  [TqCmd] -> 696MTPAIqGen/1
  Switch7/1 -> Gain1/1, Switch2/1
  696Iq_Gen_Map/1 -> Switch7/3
  Switch5/1 -> Switch1/3

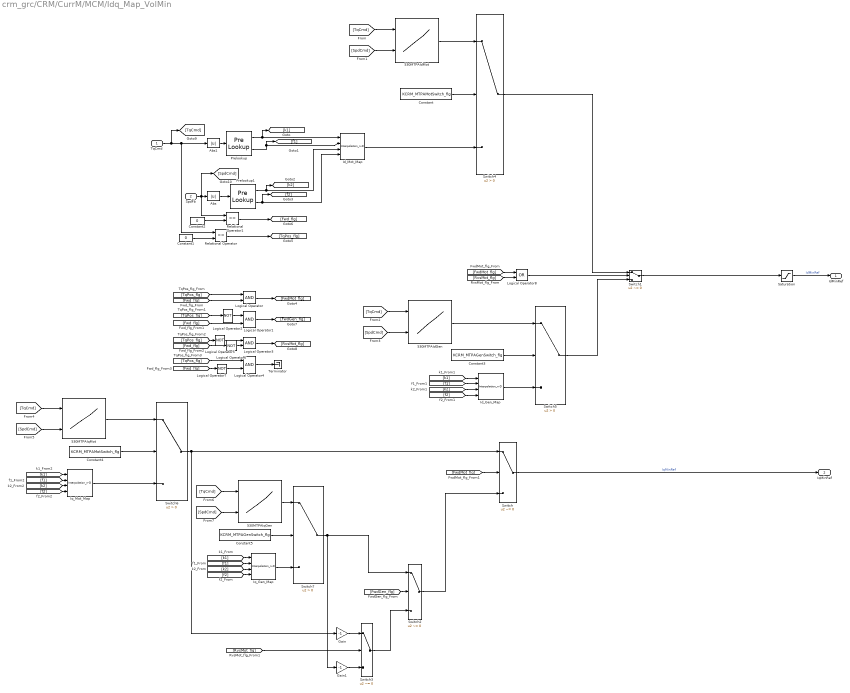
== system crm_grc/CRM/CurrM/MCM/Idq_Map_VolMin ==
  TqCmd : Inport
  SpdFb : Inport  Port=2
  530MTPAIdGen : Lookup_n-D  BreakpointsForDimension1=ACRM_MTPAIdGenMin_Y_Nm  BreakpointsForDimension2=ACRM_MTPAIdGenMin_X_rpm  Table=MCRM_MTPAIdGenMin_Z_A  InternalRulePriority=Speed  RndMeth=Simplest
      settings: InputPortMap=u0,u1
  530MTPAIdMot : Lookup_n-D  BreakpointsForDimension1=ACRM_MTPAIdMotMin_Y_Nm  BreakpointsForDimension2=ACRM_MTPAIdMotMin_X_rpm  Table=MCRM_MTPAIdMotMin_Z_A  InternalRulePriority=Speed  RndMeth=Simplest
      settings: InputPortMap=u0,u1
  530MTPAIqGen : Lookup_n-D  BreakpointsForDimension1=ACRM_MTPAIqGenMin_Y_Nm  BreakpointsForDimension2=ACRM_MTPAIqGenMin_X_rpm  Table=MCRM_MTPAIqGenMin_Z_A  InternalRulePriority=Speed  RndMeth=Simplest
      settings: InputPortMap=u0,u1
  530MTPAIqMot : Lookup_n-D  BreakpointsForDimension1=ACRM_MTPAIqMotMin_Y_Nm  BreakpointsForDimension2=ACRM_MTPAIqMotMin_X_rpm  Table=MCRM_MTPAIqMotMin_Z_A  InternalRulePriority=Speed  RndMeth=Simplest
      settings: InputPortMap=u0,u1
  Abs : Abs
  Abs1 : Abs
  Constant : Constant  Value=KCRM_MTPAMotSwitch_flg
  Constant1 : Constant  Value=0  OutDataTypeStr=uint8
  Constant2 : Constant  Value=0  OutDataTypeStr=uint8
  Constant3 : Constant  Value=KCRM_MTPAGenSwitch_flg
  Constant4 : Constant  Value=KCRM_MTPAMotSwitch_flg
  Constant5 : Constant  Value=KCRM_MTPAGenSwitch_flg
  Gain : Gain  Gain=-1
  Gain1 : Gain  Gain=-1
  Id_Gen_Map : Interpolation_n-D  Table=MCRM_MTPAIdGenMin_Z_A
  Id_Mot_Map : Interpolation_n-D  Table=MCRM_MTPAIdMotMin_Z_A
  Iq_Gen_Map : Interpolation_n-D  Table=MCRM_MTPAIqGenMin_Z_A
  Iq_Mot_Map : Interpolation_n-D  Table=MCRM_MTPAIqMotMin_Z_A
  Logical Operator{,1,3..4} (4 alike) : Logic  AllPortsSameDT=off  OutDataTypeStr=boolean
  Logical Operator{2,5..7} (4 alike) : Logic  Operator=NOT  AllPortsSameDT=off  OutDataTypeStr=boolean
  Logical Operator8 : Logic  Operator=OR  AllPortsSameDT=off  OutDataTypeStr=boolean
  Prelookup : PreLookup  BreakpointsData=ACRM_MTPAIdMotMin_Y_Nm  ExtrapMethod=Linear
  Prelookup1 : PreLookup  BreakpointsData=ACRM_MTPAIdMotMin_X_rpm  ExtrapMethod=Linear
  Relational Operator : RelationalOperator  OutDataTypeStr=boolean  InputSameDT=off
  Relational Operator1 : RelationalOperator  OutDataTypeStr=boolean  InputSameDT=off
  Saturation : Saturate  UpperLimit=0  LowerLimit=-500
      settings: AttributesFormatString=%<UpperLimit>\n%<LowerLimit>
  Switch{,1..3} (4 alike) : Switch  Criteria=u2 ~= 0
  Switch{4..7} (4 alike) : Switch  Criteria=u2 > Threshold  SaturateOnIntegerOverflow=off  InputSameDT=off
  Terminator : Terminator
  IdMinRef : Outport
  IqMinRef : Outport  Port=2
  wires:
  SpdFb/1 -> [SpdCmd], Relational Operator1/1, Abs/1
  Prelookup1/2 -> [f2], Id_Mot_Map/4
  Abs1/1 -> Prelookup/1
  Prelookup/1 -> Id_Mot_Map/1, [k1]
  [k1] -> Iq_Gen_Map/1
  Constant2/1 -> Relational Operator1/2
  [f2] -> Iq_Mot_Map/4
  Saturation/1 -> IdMinRef/1  "IdMinRef"
  Gain/1 -> Switch3/1
  Relational Operator1/1 -> [Fwd_flg]
  Logical Operator3/1 -> [RvsMot_flg]
  [TqPos_flg] -> Logical Operator2/1
  [FwdGen_flg] -> Switch2/2
  [Fwd_flg] -> Logical Operator1/2
  [f1] -> Id_Gen_Map/2
  Constant1/1 -> Relational Operator/2
  [RvsMot_flg] -> Switch3/2
  [FwdMot_flg] -> Logical Operator8/1
  Logical Operator4/1 -> Terminator/1
  Logical Operator6/1 -> Logical Operator3/2
  [Fwd_flg] -> Logical Operator7/1
  Prelookup1/1 -> [k2], Id_Mot_Map/3
  [TqPos_flg] -> Logical Operator5/1
  Prelookup/2 -> [f1], Id_Mot_Map/2
  Logical Operator2/1 -> Logical Operator1/1
  Id_Mot_Map/1 -> Switch4/3
  Abs/1 -> Prelookup1/1
  Relational Operator/1 -> [TqPos_flg]
  Switch/1 -> IqMinRef/1  "IqMinRef"
  Logical Operator1/1 -> [FwdGen_flg]
  [FwdMot_flg] -> Switch/2
  [TqPos_flg] -> Logical Operator/1
  [k1] -> Iq_Mot_Map/1
  [TqPos_flg] -> Logical Operator4/1
  [Fwd_flg] -> Logical Operator/2
  Logical Operator7/1 -> Logical Operator4/2
  Logical Operator/1 -> [FwdMot_flg]
  TqCmd/1 -> [TqCmd], Abs1/1, Relational Operator/1
  [k2] -> Iq_Mot_Map/3
  [f2] -> Iq_Gen_Map/4
  [f1] -> Iq_Gen_Map/2
  Logical Operator8/1 -> Switch1/2
  [k1] -> Id_Gen_Map/1
  [k2] -> Iq_Gen_Map/3
  Switch3/1 -> Switch2/3
  [RvsMot_flg] -> Logical Operator8/2
  [f2] -> Id_Gen_Map/4
  Gain1/1 -> Switch3/3
  [f1] -> Iq_Mot_Map/2
  [Fwd_flg] -> Logical Operator6/1
  Logical Operator5/1 -> Logical Operator3/1
  [k2] -> Id_Gen_Map/3
  Switch2/1 -> Switch/3
  Switch1/1 -> Saturation/1
  [SpdCmd] -> 530MTPAIdMot/2
  [TqCmd] -> 530MTPAIdMot/1
  [SpdCmd] -> 530MTPAIdGen/2
  [TqCmd] -> 530MTPAIdGen/1
  [SpdCmd] -> 530MTPAIqMot/2
  [TqCmd] -> 530MTPAIqMot/1
  [SpdCmd] -> 530MTPAIqGen/2
  [TqCmd] -> 530MTPAIqGen/1
  530MTPAIdMot/1 -> Switch4/1
  Constant/1 -> Switch4/2
  Switch4/1 -> Switch1/1
  Id_Gen_Map/1 -> Switch5/3
  Constant3/1 -> Switch5/2
  530MTPAIdGen/1 -> Switch5/1
  Switch5/1 -> Switch1/3
  530MTPAIqMot/1 -> Switch6/1
  Constant4/1 -> Switch6/2
  Switch6/1 -> Switch/1, Gain/1
  Iq_Mot_Map/1 -> Switch6/3
  Iq_Gen_Map/1 -> Switch7/3
  Switch7/1 -> Gain1/1, Switch2/1
  Constant5/1 -> Switch7/2
  530MTPAIqGen/1 -> Switch7/1

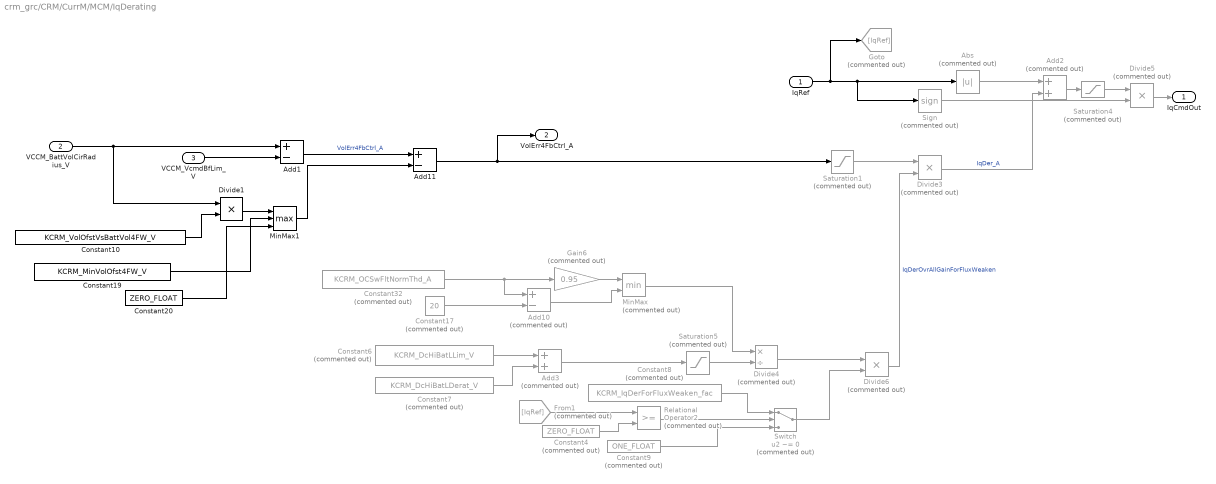
== system crm_grc/CRM/CurrM/MCM/IqDerating ==
  IqRef : Inport
  VCCM_BattVolCirRadius_V : Inport  Port=2
  VCCM_VcmdBfLim_V : Inport  Port=3
  Abs : Abs  Commented=on  SaturateOnIntegerOverflow=off
  Add1 : Sum  Inputs=+-
  Add10 : Sum  Commented=on  Inputs=+-
  Add11 : Sum  Inputs=+-
  Add2 : Sum  Commented=on
  Add3 : Sum  Commented=on
  Constant10 : Constant  Value=KCRM_VolOfstVsBattVol4FW_V  OutDataTypeStr=single
  Constant17 : Constant  Commented=on  Value=20  OutDataTypeStr=single
  Constant19 : Constant  Value=KCRM_MinVolOfst4FW_V  OutDataTypeStr=single
  Constant20 : Constant  Value=ZERO_FLOAT  OutDataTypeStr=single
  Constant32 : Constant  Commented=on  Value=KCRM_OCSwFltNormThd_A  OutDataTypeStr=single
  Constant4 : Constant  Commented=on  Value=ZERO_FLOAT  OutDataTypeStr=single
  Constant6 : Constant  Commented=on  Value=KCRM_DcHiBatLLim_V  OutDataTypeStr=single
  Constant7 : Constant  Commented=on  Value=KCRM_DcHiBatLDerat_V  OutDataTypeStr=single
  Constant8 : Constant  Commented=on  Value=KCRM_IqDerForFluxWeaken_fac  OutDataTypeStr=single
  Constant9 : Constant  Commented=on  Value=ONE_FLOAT  OutDataTypeStr=single
  Divide1 : Product  Inputs=**
  Divide3 : Product  Commented=on  Inputs=**
  Divide4 : Product  Commented=on  Inputs=*/
  Divide5 : Product  Commented=on  Inputs=**
  Divide6 : Product  Commented=on  Inputs=**
  From1 : From  Commented=on  GotoTag=IqRef
  Gain6 : Gain  Commented=on  Gain=0.95
  Goto : Goto  Commented=on  GotoTag=IqRef
  MinMax : MinMax  Commented=on  Inputs=2
  MinMax1 : MinMax  Function=max  Inputs=3
  Relational Operator2 : RelationalOperator  Commented=on  OutDataTypeStr=boolean  InputSameDT=off
  Saturation1 : Saturate  Commented=on  UpperLimit=0  LowerLimit=-inf
      settings: AttributesFormatString=%<UpperLimit>\n%<OutMax>\n%<OutMin>\n%<LowerLimit>
  Saturation4 : Saturate  Commented=on  UpperLimit=inf  LowerLimit=0
  Saturation5 : Saturate  Commented=on  UpperLimit=inf  LowerLimit=1
  Sign : Signum  Commented=on
  Switch : Switch  Commented=on  Criteria=u2 ~= 0  SaturateOnIntegerOverflow=off  InputSameDT=off
  IqCmdOut : Outport
  VolErr4FbCtrl_A : Outport  Port=2  VectorParamsAs1DForOutWhenUnconnected=off
  wires:
  Saturation5/1 -> Divide4/2
  Divide6/1 -> Divide3/2  "IqDerOvrAllGainForFluxWeaken"
  Divide4/1 -> Divide6/1
  Add3/1 -> Saturation5/1
  Constant7/1 -> Add3/2
  Constant6/1 -> Add3/1
  MinMax/1 -> Divide4/1
  Divide3/1 -> Add2/2  "IqDer_A"
  Saturation1/1 -> Divide3/1
  Constant4/1 -> Relational Operator2/2
  Relational Operator2/1 -> Switch/2
  Constant8/1 -> Switch/1
  Switch/1 -> Divide6/2
  Constant9/1 -> Switch/3
  Constant20/1 -> MinMax1/3
  Constant19/1 -> MinMax1/2
  MinMax1/1 -> Add11/2
  Divide1/1 -> MinMax1/1
  Constant10/1 -> Divide1/2
  Add1/1 -> Add11/1  "VolErr4FbCtrl_A"
  VCCM_BattVolCirRadius_V/1 -> Divide1/1, Add1/1
  VCCM_VcmdBfLim_V/1 -> Add1/2
  Add11/1 -> VolErr4FbCtrl_A/1, Saturation1/1
  Add2/1 -> Saturation4/1
  Constant32/1 -> Gain6/1, Add10/1
  Gain6/1 -> MinMax/1
  Add10/1 -> MinMax/2
  Constant17/1 -> Add10/2
  Sign/1 -> Divide5/2
  IqRef/1 -> Goto/1, Sign/1, Abs/1
  Divide5/1 -> IqCmdOut/1
  Saturation4/1 -> Divide5/1
  Abs/1 -> Add2/1
  From1/1 -> Relational Operator2/1

== system crm_grc/CRM/CurrM/MCM/IqFilter ==
  note: Description:
      | 1 order low pass filter. The constant value depends on the cut-off frequency,
  Measured : Inport  PortDimensions=1
  Add : Sum
  Constant : Constant  Value=KCRM_IqCmdFilCoeff_null  OutDataTypeStr=single
  Product : Product  RndMeth=Zero
  Subtract : Sum  Inputs=+-
  Unit Delay : UnitDelay  SampleTime=-1
  Filtered : Outport
  wires:
  Add/1 -> Unit Delay/1, Filtered/1
  Product/1 -> Add/1
  Constant/1 -> Product/2
  Subtract/1 -> Product/1
  Unit Delay/1 -> Add/2, Subtract/2
  Measured/1 -> Subtract/1

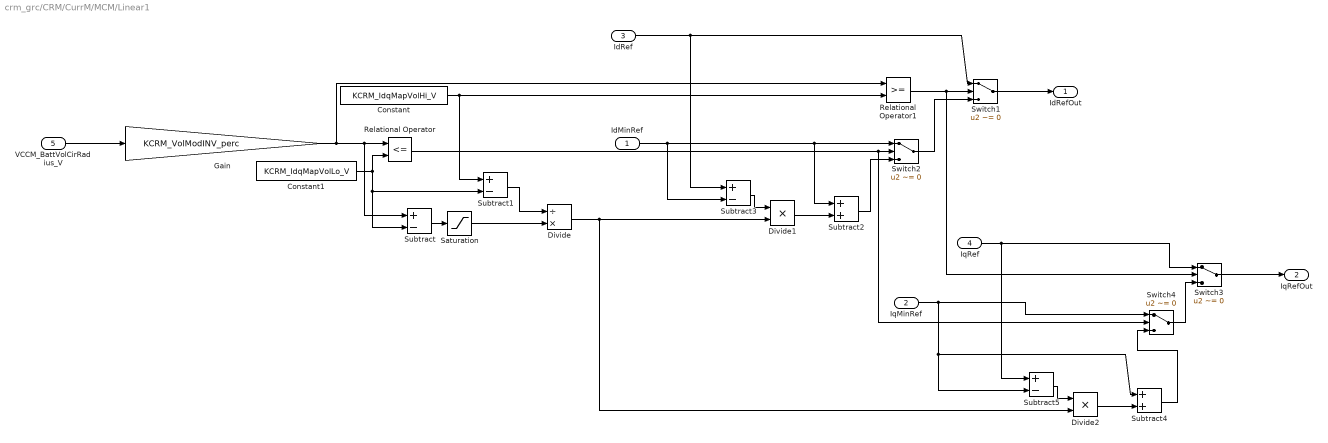
== system crm_grc/CRM/CurrM/MCM/Linear1 ==
  IdMinRef : Inport
  IqMinRef : Inport  Port=2
  IdRef : Inport  Port=3
  IqRef : Inport  Port=4
  VCCM_BattVolCirRadius_V : Inport  Port=5
  Constant : Constant  Value=KCRM_IdqMapVolHi_V  OutDataTypeStr=single
  Constant1 : Constant  Value=KCRM_IdqMapVolLo_V  OutDataTypeStr=single
  Divide : Product  Inputs=/*
  Divide1 : Product  Inputs=**
  Divide2 : Product  Inputs=**
  Gain : Gain  Gain=KCRM_VolModINV_perc
  Relational Operator : RelationalOperator  Operator=<=  OutDataTypeStr=boolean  InputSameDT=off
  Relational Operator1 : RelationalOperator  OutDataTypeStr=boolean  InputSameDT=off
  Saturation : Saturate  UpperLimit=inf  LowerLimit=0.5
  Subtract{,1,3,5} (4 alike) : Sum  Inputs=+-
  Subtract2 : Sum
  Subtract4 : Sum
  Switch{1..4} (4 alike) : Switch  Criteria=u2 ~= 0  SaturateOnIntegerOverflow=off  InputSameDT=off
  IdRefOut : Outport
  IqRefOut : Outport  Port=2
  wires:
  VCCM_BattVolCirRadius_V/1 -> Gain/1
  Gain/1 -> Relational Operator1/1, Relational Operator/1, Subtract/1
  Constant1/1 -> Relational Operator/2, Subtract/2, Subtract1/2
  Constant/1 -> Relational Operator1/2, Subtract1/1
  Relational Operator1/1 -> Switch1/2, Switch3/2
  IdRef/1 -> Switch1/1, Subtract3/1
  Relational Operator/1 -> Switch2/2, Switch4/2
  Switch2/1 -> Switch1/3
  Switch1/1 -> IdRefOut/1
  IdMinRef/1 -> Switch2/1, Subtract2/1, Subtract3/2
  Subtract/1 -> Saturation/1
  Subtract1/1 -> Divide/1
  Divide/1 -> Divide1/2, Divide2/2
  Divide1/1 -> Subtract2/2
  Subtract3/1 -> Divide1/1
  Subtract2/1 -> Switch2/3
  Saturation/1 -> Divide/2
  IqRef/1 -> Switch3/1, Subtract5/1
  Switch3/1 -> IqRefOut/1
  Switch4/1 -> Switch3/3
  IqMinRef/1 -> Switch4/1, Subtract4/1, Subtract5/2
  Divide2/1 -> Subtract4/2
  Subtract5/1 -> Divide2/1
  Subtract4/1 -> Switch4/3

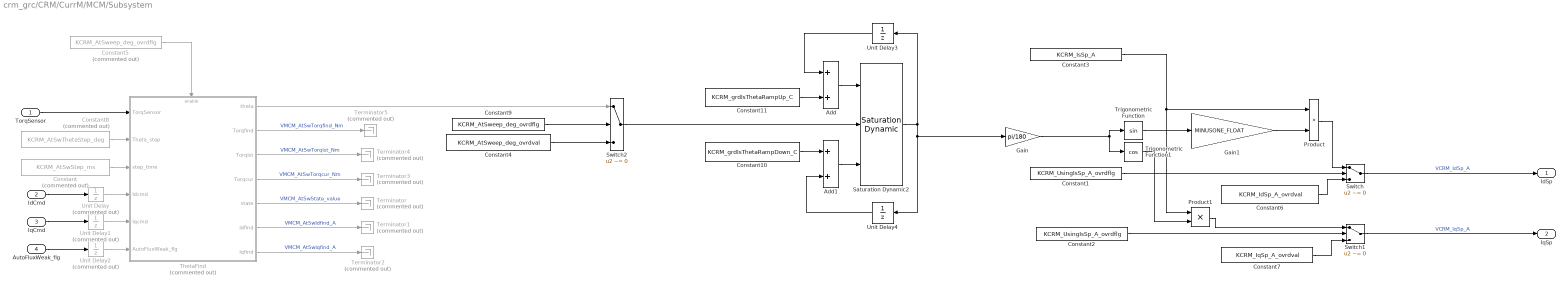
== system crm_grc/CRM/CurrM/MCM/Subsystem ==
  "TorqSensor " : Inport
  "IdCmd " : Inport  Port=2
  "IqCmd " : Inport  Port=3
  "AutoFluxWeak_flg " : Inport  Port=4
  Add : Sum
  Add1 : Sum
  Constant : Constant  Commented=on  Value=KCRM_AtSwStep_ms  OutDataTypeStr=int32
  Constant1 : Constant  Value=KCRM_UsingIsSp_A_ovrdflg  OutDataTypeStr=single
  Constant10 : Constant  Value=KCRM_grdIsThetaRampDown_C
  Constant11 : Constant  Value=KCRM_grdIsThetaRampUp_C
  Constant2 : Constant  Value=KCRM_UsingIsSp_A_ovrdflg  OutDataTypeStr=single
  Constant3 : Constant  Value=KCRM_IsSp_A  OutDataTypeStr=single
  Constant4 : Constant  Value=KCRM_AtSweep_deg_ovrdval  OutDataTypeStr=single
  Constant5 : Constant  Commented=on  Value=KCRM_AtSweep_deg_ovrdflg  OutDataTypeStr=single
  Constant6 : Constant  Value=KCRM_IdSp_A_ovrdval  OutDataTypeStr=single
  Constant7 : Constant  Value=KCRM_IqSp_A_ovrdval  OutDataTypeStr=single
  Constant8 : Constant  Commented=on  Value=KCRM_AtSwThetaStep_deg  OutDataTypeStr=single
  Constant9 : Constant  Value=KCRM_AtSweep_deg_ovrdflg  OutDataTypeStr=single
  Gain : Gain  Gain=pi/180
  Gain1 : Gain  Gain=MINUSONE_FLOAT
  Product : Product  RndMeth=Zero
  Product1 : Product  RndMeth=Zero
  Saturation Dynamic2 : simulink/Discontinuities/Saturation Dynamic  OutMin=[]  OutMax=[]  OutDataTypeStr=Inherit: Same as second input  OutDataType=fixdt(1, 16)  OutScaling=2^-10  DoSatur=off
  Switch : Switch  Criteria=u2 ~= 0  SaturateOnIntegerOverflow=off  InputSameDT=off
  Switch1 : Switch  Criteria=u2 ~= 0  SaturateOnIntegerOverflow=off  InputSameDT=off
  Switch2 : Switch  Criteria=u2 ~= 0  SaturateOnIntegerOverflow=off  InputSameDT=off
  Terminator{,1..5} (6 alike) : Terminator  Commented=on
  ThetaFind : Subsystem  Commented=on
  Trigonometric Function : Trigonometry
  Trigonometric Function1 : Trigonometry  Operator=cos
  Unit Delay : UnitDelay  Commented=on  SampleTime=-1  HasFrameUpgradeWarning=on
  Unit Delay1 : UnitDelay  Commented=on  SampleTime=-1  HasFrameUpgradeWarning=on
  Unit Delay2 : UnitDelay  Commented=on  SampleTime=-1  HasFrameUpgradeWarning=on
  Unit Delay3 : UnitDelay  SampleTime=-1  HasFrameUpgradeWarning=on
  Unit Delay4 : UnitDelay  SampleTime=-1  HasFrameUpgradeWarning=on
  IdSp : Outport
  IqSp : Outport  Port=2
  wires:
  Switch/1 -> IdSp/1  "VCRM_IdSp_A"
  Constant6/1 -> Switch/3
  Constant1/1 -> Switch/2
  Constant2/1 -> Switch1/2
  Constant7/1 -> Switch1/3
  Switch1/1 -> IqSp/1  "VCRM_IqSp_A"
  Constant3/1 -> Product1/1, Product/1
  Gain/1 -> Trigonometric Function/1, Trigonometric Function1/1
  Trigonometric Function/1 -> Gain1/1
  Product/1 -> Switch/1
  Product1/1 -> Switch1/1
  Trigonometric Function1/1 -> Product1/2
  Gain1/1 -> Product/2
  Constant5/1 -> ThetaFind/Enable
  "TorqSensor "/1 -> ThetaFind/1(TorqSensor)
  Constant/1 -> ThetaFind/3(step_time)
  Constant8/1 -> ThetaFind/2(Theta_step)
  ThetaFind/5(state) -> Terminator/1  "VMCM_AtSwState_value"
  ThetaFind/6(Idfind) -> Terminator1/1  "VMCM_AtSwIdfind_A"
  ThetaFind/7(Iqfind) -> Terminator2/1  "VMCM_AtSwIqfind_A"
  Constant9/1 -> Switch2/2
  ThetaFind/1(theta) -> Switch2/1
  Unit Delay/1 -> ThetaFind/4(Idcmd)
  Unit Delay1/1 -> ThetaFind/5(Iqcmd)
  ThetaFind/4(Torqcur) -> Terminator3/1  "VMCM_AtSwTorqcur_Nm"
  ThetaFind/3(Torqlst) -> Terminator4/1  "VMCM_AtSwTorqlst_Nm"
  ThetaFind/2(Torqfind) -> Terminator5/1  "VMCM_AtSwTorqfind_Nm"
  "IdCmd "/1 -> Unit Delay/1
  "IqCmd "/1 -> Unit Delay1/1
  "AutoFluxWeak_flg "/1 -> Unit Delay2/1
  Unit Delay2/1 -> ThetaFind/6("AutoFluxWeak_flg ")
  Constant4/1 -> Switch2/3
  Add1/1 -> Saturation Dynamic2/3
  Switch2/1 -> Saturation Dynamic2/2
  Unit Delay4/1 -> Add1/2
  Saturation Dynamic2/1 -> Gain/1, Unit Delay4/1, Unit Delay3/1
  Constant11/1 -> Add/2
  Constant10/1 -> Add1/1
  Add/1 -> Saturation Dynamic2/1
  Unit Delay3/1 -> Add/1

== system crm_grc/CRM/CurrM/MCM/Subsystem1 ==
  Constant1 : Constant  Value=KMCM_UsingIsSp_flg  OutDataTypeStr=single
  Constant2 : Constant  Value=KMCM_UsingIsSp_flg  OutDataTypeStr=single
  Constant3 : Constant  Value=KMCM_IsSp_A  OutDataTypeStr=single
  Constant4 : Constant  Value=KMCM_IsTheta_deg  OutDataTypeStr=single
  Constant6 : Constant  Value=KMCM_IdSp_A  OutDataTypeStr=single
  Constant7 : Constant  Value=KMCM_IqSp_A  OutDataTypeStr=single
  Gain : Gain  Gain=pi/180
  Gain1 : Gain  Gain=-1
  Product : Product  RndMeth=Zero
  Product1 : Product  RndMeth=Zero
  Switch : Switch  Criteria=u2 ~= 0  SaturateOnIntegerOverflow=off  InputSameDT=off
  Switch1 : Switch  Criteria=u2 ~= 0  SaturateOnIntegerOverflow=off  InputSameDT=off
  ThetaFind : Subsystem
  Trigonometric Function : Trigonometry
  Trigonometric Function1 : Trigonometry  Operator=cos
  IdSp : Outport
  IqSp : Outport  Port=2
  wires:
  Gain1/1 -> Product/2
  Trigonometric Function1/1 -> Product1/2
  Product1/1 -> Switch1/1
  Product/1 -> Switch/1
  Trigonometric Function/1 -> Gain1/1
  Gain/1 -> Trigonometric Function1/1, Trigonometric Function/1
  Constant4/1 -> Gain/1
  Constant3/1 -> Product1/1, Product/1
  Switch1/1 -> IqSp/1
  Constant7/1 -> Switch1/3
  Constant2/1 -> Switch1/2
  Constant1/1 -> Switch/2
  Constant6/1 -> Switch/3
  Switch/1 -> IdSp/1

== system crm_grc/CRM/CurrM/MCM/FluxWeaken /PI  ==
  error : Inport
  Kp : Inport  Port=2
  Ki : Inport  Port=3
  Lower Limit : Inport  Port=4
  "Reset " : Inport  Port=5
  Anti-windup : Subsystem
  Constant : Constant  Value=ZERO_FLOAT  OutDataTypeStr=Inherit: Inherit via back propagation
  Discrete-Time Integrator : DiscreteIntegrator  IntegratorMethod=Accumulation: Forward Euler  ExternalReset=level  SampleTime=-1  ICPrevOutput=DiscIntNeverNeededParam  ICPrevScaledInput=DiscIntNeverNeededParam
  Product : Product  RndMeth=Simplest  OutDataTypeStr=Inherit: Same as first input
  Product1 : Product  RndMeth=Simplest  OutDataTypeStr=Inherit: Same as first input
  Saturation Dynamic : simulink/Discontinuities/Saturation Dynamic  OutMin=[]  OutMax=[]  OutDataTypeStr=Inherit: Same as second input  OutDataType=fixdt(1, 16)  OutScaling=2^-10  RndMeth=Simplest  DoSatur=off
  Sum : Sum  Inputs=|++  RndMeth=Simplest  SaturateOnIntegerOverflow=on  OutDataTypeStr=Inherit: Same as first input
  Out : Outport
  wires:
  Lower Limit/1 -> Anti-windup/4(Lower Limit), Saturation Dynamic/3
  error/1 -> Product1/2, Product/1
  Kp/1 -> Product1/1
  Ki/1 -> Product/2
  Sum/1 -> Anti-windup/2(preSat), Saturation Dynamic/2
  Product/1 -> Anti-windup/1(preInt)
  Product1/1 -> Sum/1
  Constant/1 -> Anti-windup/3(Upper Limit), Saturation Dynamic/1
  Saturation Dynamic/1 -> Out/1
  Anti-windup/1(Out) -> Discrete-Time Integrator/1
  Discrete-Time Integrator/1 -> Sum/2
  "Reset "/1 -> Discrete-Time Integrator/2

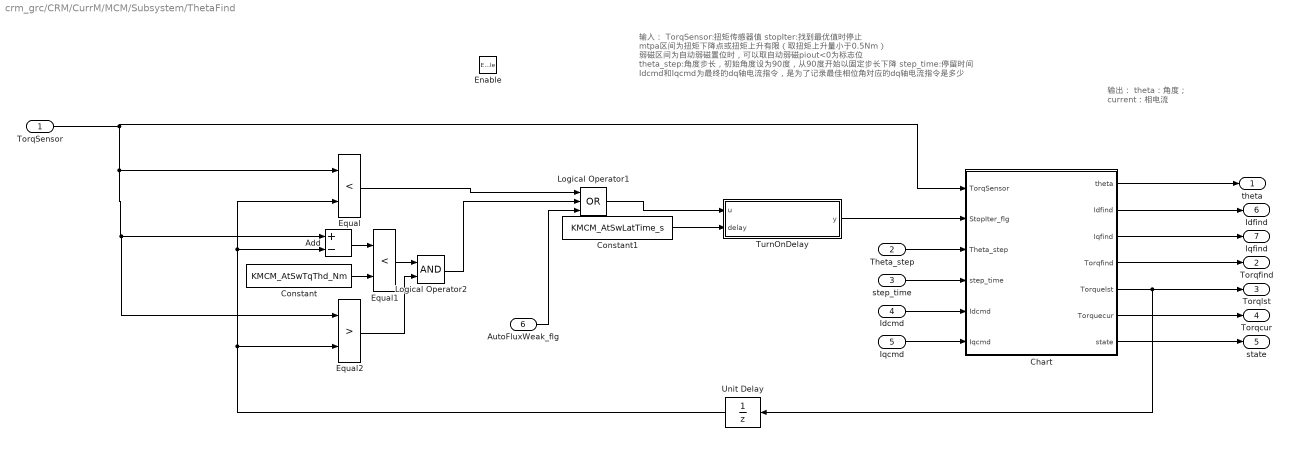
== system crm_grc/CRM/CurrM/MCM/Subsystem/ThetaFind ==
  note: 输入：
      | TorqSensor:扭矩传感器值
      | stopIter:找到最优值时停止 mtpa区间为扭矩下降点或扭矩上升有限（取扭矩上升量小于0.5Nm） 弱磁区间为自动弱磁置位时，可以取自动弱磁piout<0为标志位
      | theta_step:角度步长，初始角度设为90度，从90度开始以固定步长下降
      | step_time:停留时间
      | Idcmd和Iqcmd为最终的dq轴电流指令，是为了记录最佳相位角对应的dq轴电流指令是多少
  note: 输出：
      | theta：角度；
      | current：相电流
  TorqSensor : Inport
  Theta_step : Inport  Port=2
  step_time : Inport  Port=3
  Idcmd : Inport  Port=4
  Iqcmd : Inport  Port=5
  "AutoFluxWeak_flg " : Inport  Port=6
  Enable : EnablePort  StatesWhenEnabling=reset
  Add : Sum  Inputs=+-
  Chart : Stateflow chart  TreatAsAtomicUnit=on
  Constant : Constant  Value=KMCM_AtSwTqThd_Nm
  Constant1 : Constant  Value=KMCM_AtSwLatTime_s  OutDataTypeStr=single
  Equal : RelationalOperator  Operator=<  OutDataTypeStr=boolean  RndMeth=Simplest  InputSameDT=off
  Equal1 : RelationalOperator  Operator=<  OutDataTypeStr=boolean  RndMeth=Simplest  InputSameDT=off
  Equal2 : RelationalOperator  Operator=>  OutDataTypeStr=boolean  RndMeth=Simplest  InputSameDT=off
  Logical Operator1 : Logic  Operator=OR  Inputs=3  AllPortsSameDT=off  OutDataTypeStr=boolean
  Logical Operator2 : Logic  AllPortsSameDT=off  OutDataTypeStr=boolean
  TurnOnDelay : Subsystem  AncestorBlock=Legion_lib/Logic Blocks/TurnOnDelay
      mask Display:
      | color('red');
      | disp('Turn On Delay')
  Unit Delay : UnitDelay  SampleTime=-1  HasFrameUpgradeWarning=on
  theta : Outport  VectorParamsAs1DForOutWhenUnconnected=off
  Torqfind : Outport  Port=2  VectorParamsAs1DForOutWhenUnconnected=off
  Torqlst : Outport  Port=3  VectorParamsAs1DForOutWhenUnconnected=off
  Torqcur : Outport  Port=4  VectorParamsAs1DForOutWhenUnconnected=off
  state : Outport  Port=5  VectorParamsAs1DForOutWhenUnconnected=off
  Idfind : Outport  Port=6  VectorParamsAs1DForOutWhenUnconnected=off
  Iqfind : Outport  Port=7  VectorParamsAs1DForOutWhenUnconnected=off
  wires:
  step_time/1 -> Chart/4(step_time)
  Theta_step/1 -> Chart/3(Theta_step)
  TorqSensor/1 -> Equal/1, Equal2/1, Add/1, Chart/1(TorqSensor)
  Chart/1(theta) -> theta/1
  Chart/2(Idfind) -> Idfind/1
  Chart/3(Iqfind) -> Iqfind/1
  Idcmd/1 -> Chart/5(Idcmd)
  Iqcmd/1 -> Chart/6(Iqcmd)
  Equal/1 -> Logical Operator1/1
  Chart/4(Torqfind) -> Torqfind/1
  Add/1 -> Equal1/1
  Constant/1 -> Equal1/2
  Equal1/1 -> Logical Operator2/1
  Equal2/1 -> Logical Operator2/2
  Logical Operator2/1 -> Logical Operator1/2
  Chart/5(Torquelst) -> Unit Delay/1, Torqlst/1
  Chart/6(Torquecur) -> Torqcur/1
  Chart/7(state) -> state/1
  Constant1/1 -> TurnOnDelay/2(delay)
  TurnOnDelay/1(y) -> Chart/2(StopIter_flg)
  Logical Operator1/1 -> TurnOnDelay/1(u)
  "AutoFluxWeak_flg "/1 -> Logical Operator1/3
  Unit Delay/1 -> Equal2/2, Add/2, Equal/2
